simulink model "practica11"  (R2015a)
settings: Solver=ode45  StartTime=0.0  StopTime=30  RelTol=1e-3
values from neighbouring files (symbols this model uses):
  b = 1    [practica11cc.m]    (also in practica12.m; practica13.m; practica16.m; practica17.m)
  d = .1    (= 0.1)    [practica11cc.m]    (also in practica20upiita.m = 1)
  k = 1    [practica11cc.m]    (also in practica12.m; practica16.m; practica17.m; practica22.m)
  k1 = 1    [practica10cc.m]    (also in practica11cc.m = 2; practica24.m = 5.0759)
  l = 1    [practica11cc.m]    (also in practica13.m; practica17.m; practica18.m; practica26.m)
  m = 1    [practica11cc.m]    (also in practica12.m; practica13.m; practica16.m; practica17.m)
  r = 1    [practica11cc.m]    (also in practica19.m = 0.5; practica34.m = roots([1 11 44 34+k]); practica4.m; practica6cc.m)
settings Model: Creator=Sala7  LastModifiedBy=Sala7

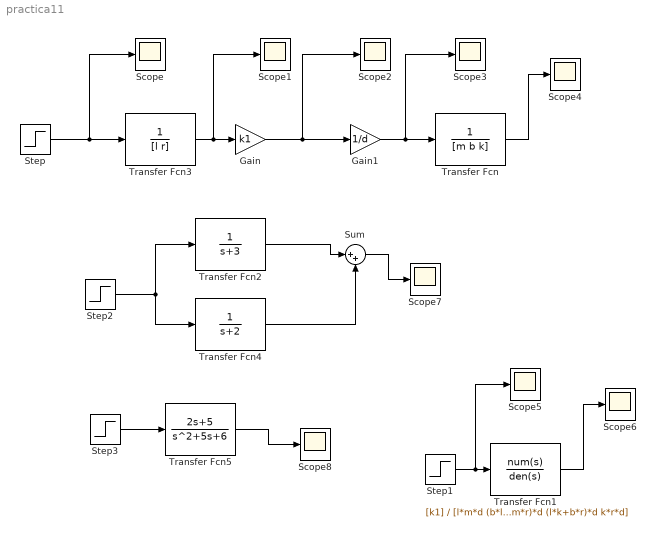
== system practica11 ==
  Gain : Gain  Gain=k1
  Gain1 : Gain  Gain=1/d
  Scope{,1..8} (9 alike) : Scope
      Scope2 settings: SaveName=ScopeData2
      Scope3 settings: SaveName=ScopeData3
      Scope4 settings: SaveName=ScopeData4
      Scope5 settings: SaveName=ScopeData5
      Scope6 settings: SaveName=ScopeData6
      Scope7 settings: SaveName=ScopeData7
      Scope8 settings: SaveName=ScopeData8
  Step{,1..3} (4 alike) : Step  SampleTime=0
  Sum : Sum  Inputs=|++
  Transfer Fcn : TransferFcn  Denominator=[m b k]
  Transfer Fcn1 : TransferFcn  Numerator=[k1]  Denominator=[l*m*d (b*l+m*r)*d (l*k+b*r)*d k*r*d]
  Transfer Fcn2 : TransferFcn  Denominator=[1 3]
  Transfer Fcn3 : TransferFcn  Denominator=[l r]
  Transfer Fcn4 : TransferFcn  Denominator=[1 2]
  Transfer Fcn5 : TransferFcn  Numerator=[2 5]  Denominator=[1 5 6]
  wires:
  Transfer Fcn3/1 -> Scope1/1, Gain/1
  Gain/1 -> Scope2/1, Gain1/1
  Gain1/1 -> Scope3/1, Transfer Fcn/1
  Step/1 -> Scope/1, Transfer Fcn3/1
  Transfer Fcn/1 -> Scope4/1
  Step1/1 -> Scope5/1, Transfer Fcn1/1
  Transfer Fcn1/1 -> Scope6/1
  Transfer Fcn2/1 -> Sum/1
  Transfer Fcn4/1 -> Sum/2
  Step2/1 -> Transfer Fcn4/1, Transfer Fcn2/1
  Sum/1 -> Scope7/1
  Step3/1 -> Transfer Fcn5/1
  Transfer Fcn5/1 -> Scope8/1
